simulink model "data_parametric_model_block"  (R2015a)
settings: Solver=ode45  StartTime=0.0  StopTime=10.0  RelTol=1e-3
libraries: simulink x4, RCTblocks x1
settings Model: CovSFcnEnable=off  Creator=scorpii  LastModifiedBy=shawn
settings OptimizationCC: BlockReduction=off  InlineParams=on  BufferReuse=off
settings DebuggingCC: SolverPrmCheckMsg=warning

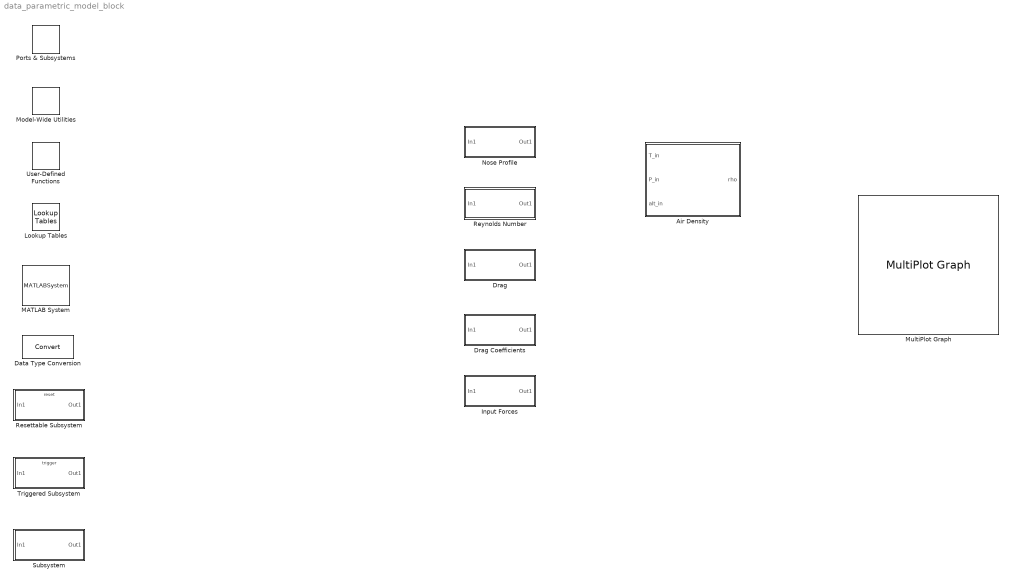
== system data_parametric_model_block ==
  Air Density : MATLAB Function  TreatAsAtomicUnit=on
  Data Type Conversion : DataTypeConversion
  Drag : Subsystem
  Drag Coefficients : Subsystem
  Input Forces : Subsystem
  Lookup Tables : simulink/Lookup Tables  SystemSampleTime=-1
  MATLAB System : MATLABSystem
  Model-Wide Utilities : simulink/Model-Wide Utilities  SystemSampleTime=-1
  MultiPlot Graph : RCTblocks/MultiPlot Graph  Tag=MultiPlot  tmin=0  tmax=20  ymin=-1  ymax=1  Tsamp=-1  vnamesave=multisimout
  Nose Profile : Subsystem
  Ports & Subsystems : simulink/Ports & Subsystems  SystemSampleTime=-1
  Resettable Subsystem : Subsystem  TreatAsAtomicUnit=on
  Reynolds Number : Subsystem
  Subsystem : Subsystem
  Triggered Subsystem : Subsystem  TreatAsAtomicUnit=on
  User-Defined Functions : simulink/User-Defined Functions  SystemSampleTime=-1
      link override "MATLAB Function/ Demux ": Outputs=1
      link override "MATLAB Function/ SFunction ": FunctionName=sf_sfun
      link override MATLAB Function/u: Port=1
      link override MATLAB Function/y: Port=1

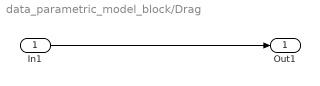
== system data_parametric_model_block/Drag ==
  In1 : Inport
  Out1 : Outport
  wires:
  In1/1 -> Out1/1

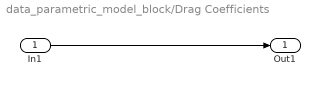
== system data_parametric_model_block/Drag Coefficients ==
  In1 : Inport
  Out1 : Outport
  wires:
  In1/1 -> Out1/1

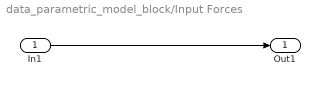
== system data_parametric_model_block/Input Forces ==
  In1 : Inport
  Out1 : Outport
  wires:
  In1/1 -> Out1/1

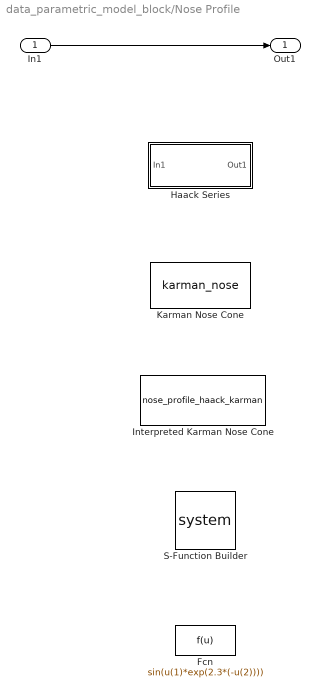
== system data_parametric_model_block/Nose Profile ==
  In1 : Inport
  Fcn : Fcn  Expr=sin(u(1)*exp(2.3*(-u(2))))
  Haack Series : Subsystem
  Interpreted Karman Nose Cone : MATLABFcn  MATLABFcn=nose_profile_haack_karman
  Karman Nose Cone : S-Function  FunctionName=karman_nose
  S-Function Builder : S-Function  mask(S-Function Builder){}
      mask help: Simulink:masks:SFunctionBuilder_MD
      mask init:
      | val = [[.9  0.75 0.75 1 1 .9 .9 1]',[1 1 0.75 0.75 .9 .9 1 .9]'];try , sys = get_param(gcb,'SfunBuilderFcnName');if isempty(sys), sys = get_param(gcb,'FunctionName'); end,catch, sys = get_param(gcb,'FunctionName'); end
      settings: CopyFcn=set_param(gcbh,'LinkStatus','none')  OpenFcn=sfunctionwizard(gcbh)
      mask Display: plot(val(:,1),val(:,2)),disp(sys), port_label('input',1,'u0'), port_label('output',1,'y0')
  Out1 : Outport
  wires:
  In1/1 -> Out1/1

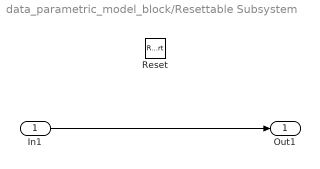
== system data_parametric_model_block/Resettable Subsystem ==
  In1 : Inport
  Reset : ResetPort  DisableCoverage=on
  Out1 : Outport
  wires:
  In1/1 -> Out1/1

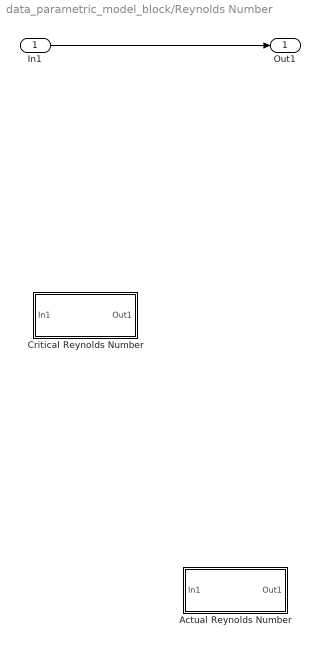
== system data_parametric_model_block/Reynolds Number ==
  In1 : Inport
  Actual Reynolds Number : Subsystem
  Critical Reynolds Number : Subsystem
  Out1 : Outport
  wires:
  In1/1 -> Out1/1

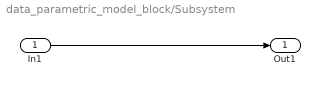
== system data_parametric_model_block/Subsystem ==
  In1 : Inport
  Out1 : Outport
  wires:
  In1/1 -> Out1/1

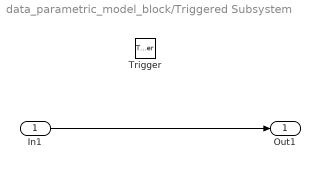
== system data_parametric_model_block/Triggered Subsystem ==
  In1 : Inport
  Trigger : TriggerPort
  Out1 : Outport
  wires:
  In1/1 -> Out1/1

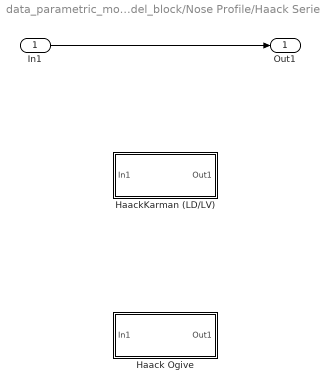
== system data_parametric_model_block/Nose Profile/Haack Series ==
  In1 : Inport
  Haack Ogive : Subsystem
  HaackKarman (LD/LV) : Subsystem
  Out1 : Outport
  wires:
  In1/1 -> Out1/1

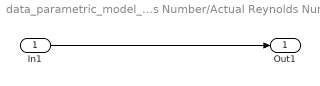
== system data_parametric_model_block/Reynolds Number/Actual Reynolds Number ==
  In1 : Inport
  Out1 : Outport
  wires:
  In1/1 -> Out1/1

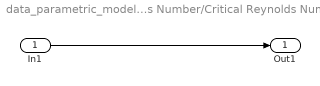
== system data_parametric_model_block/Reynolds Number/Critical Reynolds Number ==
  In1 : Inport
  Out1 : Outport
  wires:
  In1/1 -> Out1/1

== system data_parametric_model_block/Nose Profile/Haack Series/Haack Ogive ==
  In1 : Inport
  Out1 : Outport
  wires:
  In1/1 -> Out1/1

== system data_parametric_model_block/Nose Profile/Haack Series/HaackKarman (LD//LV) ==
  In1 : Inport
  Out1 : Outport
  wires:
  In1/1 -> Out1/1

== matlab function data_parametric_model_block/User-Defined Functions/MATLAB Function ==
  data: u input; y output
function y = fcn(u)
%#codegen

y = u;

== matlab function data_parametric_model_block/Air Density ==
  data: T_in input; rho output; P_in input; alt_in input
function rho = ISA_model(T_in, P_in, alt_in)

% This model computes the gas characteristics of the atmosphere around the
% rocket based on temperature and pressure at launch and current altitude.
% It uses the International Standard Atmosphere (ISA) model. This model is 
% only effective BELOW the tropopause.

% Model is based on the following document:
%   http://home.anadolu.edu.tr/~mcavcar/common/ISAweb.pdf

% Define required constants for the model as per ISA mean sea-level
% conditions:
%   P_o     = standard pressure (Pascals)
%   T_o     = standard temperature (degrees K)
%   R       = gas Constants (m^2/K*s^2)

    P_o     = 101325;
    T_o     = 288.15;
    R       = 287.04;
    
% The following recalculates the temperature in terms of ISA deviation.
% Variables used:
%   T_dev   = ISA deviation temperature (degrees C)
%   T_in    = ground temperature (degrees C)

    T_dev   = T_in - T_o + 273.15;
    
% The following calculates the temperature at the current altitude.
% Variables used:
%   T_act   = Actual temperature at current altitude (degrees K)
%   alt_in  = Actual altitude (m)

    T_act   = (T_o + T_dev) - (6.5/1000)*alt_in;
    
% The following recalculates the pressure in terms of ISA deviation.
% Variables used:
%   P_dev   = ISA deviation pressure (Pascals)
%   P_in    = ground pressure (Pascals)

    P_dev   = P_in - P_o;
    
% The following calculates the ambient pressure at the current altitude.
% Variables used:
%   P_act   = actual pressure at current altitude (Pascals)

    P_act   = (P_o + P_dev)*((1 - 0.0065*(alt_in/(T_o + T_dev)))^5.2561);
    
% The following calculates the air density at the current altitude.
% Variables used:
%   rho = air density at current altitude (Kg/m^3)

    rho = P_act/(R*T_act);
    
% END OF FUNCTION
